simulink model "Final_Project_Ball_Beam_SimulinkModel"  (R2017b)
settings: Solver=ode45  StartTime=0.0  StopTime=10.0  RelTol=1e-3
undefined symbols (not defined in the file): d, g, J, L, m, r
settings Model: Creator=sansh  LastModifiedBy=green
settings CodeAppCC: StateflowObjectComments=on

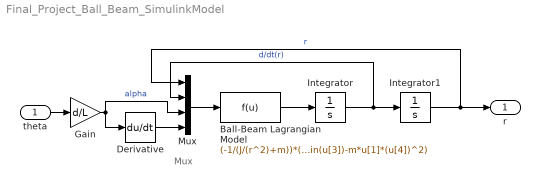
== system Final_Project_Ball_Beam_SimulinkModel ==
  note: Mux
  theta : Inport
  Ball-Beam Lagrangian Model : Fcn  Expr=(-1/(J/(r^2)+m))*(m*g*sin(u[3])-m*u[1]*(u[4])^2)
  Derivative : Derivative
  Gain : Gain  Gain=d/L
  Integrator : Integrator
  Integrator1 : Integrator
  Mux : Mux
  r : Outport
  wires:
  Integrator/1 -> Mux/2, Integrator1/1  "d/dt(r)"
  Integrator1/1 -> Mux/1, r/1  "r"
  Ball-Beam Lagrangian Model/1 -> Integrator/1
  Mux/1 -> Ball-Beam Lagrangian Model/1
  theta/1 -> Gain/1
  Gain/1 -> Derivative/1, Mux/3  "alpha"
  Derivative/1 -> Mux/4
